simulink model "reaktor_s"  (R2016a)
settings: Solver=VariableStepAuto  StartTime=0.0  StopTime=100  RelTol=1e-3
settings Model: Creator=Michal Chruscinski  LastModifiedBy=Michal Chruscinski

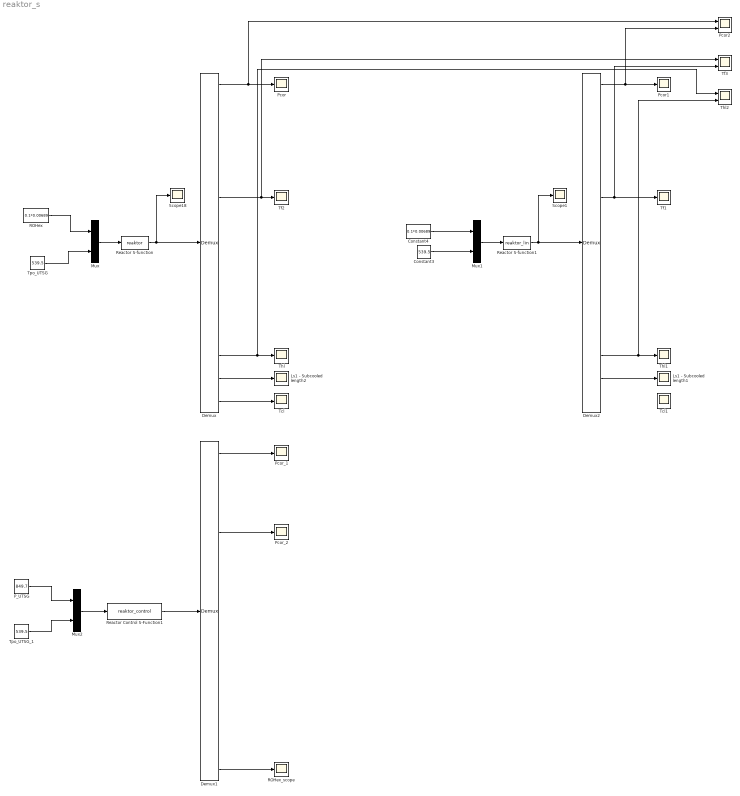
== system reaktor_s ==
  Constant3 : Constant  Value=539.5
  Constant4 : Constant  Value=0.1*0.00689
  Demux : Demux  Outputs=15
  Demux1 : Demux  Outputs=21
  Demux2 : Demux  Outputs=15
  Ls1 - Subcooled length1 : Scope
  Ls1 - Subcooled length2 : Scope
  Mux : Mux  Inputs=2
  Mux1 : Mux  Inputs=2
  Mux2 : Mux  Inputs=2
  P_UTSG : Constant  Value=849.7
  Pcor : Scope
  Pcor1 : Scope
  Pcor2 : Scope  NumInputPorts=2
  Pcor_1 : Scope
  Pcor_2 : Scope
  ROHex : Constant  Value=0.1*0.00689
  ROHex_scope : Scope
  Reactor Control S-Function1 : S-Function  FunctionName=reaktor_control  SFunctionDeploymentMode=off  EnableBusSupport=off
  Reactor S-function : S-Function  FunctionName=reaktor  SFunctionDeploymentMode=off  EnableBusSupport=off
  Reactor S-function1 : S-Function  FunctionName=reaktor_lin  SFunctionDeploymentMode=off  EnableBusSupport=off
  Scope1 : Scope
  Scope18 : Scope
  Tcl : Scope
  Tcl1 : Scope
  Tf1 : Scope
  Tf2 : Scope
  Tf3 : Scope  NumInputPorts=2
  Thl : Scope
  Thl1 : Scope
  Thl2 : Scope  NumInputPorts=2
  Tpo_UTSG : Constant  Value=539.5
  Tpo_UTSG_1 : Constant  Value=539.5
  wires:
  Demux/1 -> Pcor2/1, Pcor/1
  Reactor S-function/1 -> Scope18/1, Demux/1
  Tpo_UTSG/1 -> Mux/2
  Mux/1 -> Reactor S-function/1
  Demux/6 -> Tf3/1, Tf2/1
  Demux/14 -> Ls1 - Subcooled length2/1
  Demux/15 -> Tcl/1
  Demux/13 -> Thl2/1, Thl/1
  ROHex/1 -> Mux/1
  Mux2/1 -> Reactor Control S-Function1/1
  P_UTSG/1 -> Mux2/1
  Tpo_UTSG_1/1 -> Mux2/2
  Reactor Control S-Function1/1 -> Demux1/1
  Demux1/1 -> Pcor_1/1
  Demux1/21 -> ROHex_scope/1
  Demux1/6 -> Pcor_2/1
  Demux2/1 -> Pcor2/2, Pcor1/1
  Reactor S-function1/1 -> Scope1/1, Demux2/1
  Constant3/1 -> Mux1/2
  Mux1/1 -> Reactor S-function1/1
  Demux2/6 -> Tf1/1, Tf3/2
  Demux2/14 -> Ls1 - Subcooled length1/1
  Demux2/13 -> Thl2/2, Thl1/1
  Constant4/1 -> Mux1/1
